simulink model "model_5modes"  (R2020a)
settings: Solver=VariableStepAuto  StartTime=0.0  StopTime=Inf  RelTol=1e-3
libraries: dspobslib x1
settings Model: Creator=Dinh-Viet-Toan  LastModifiedBy=Dinh-Viet-Toan

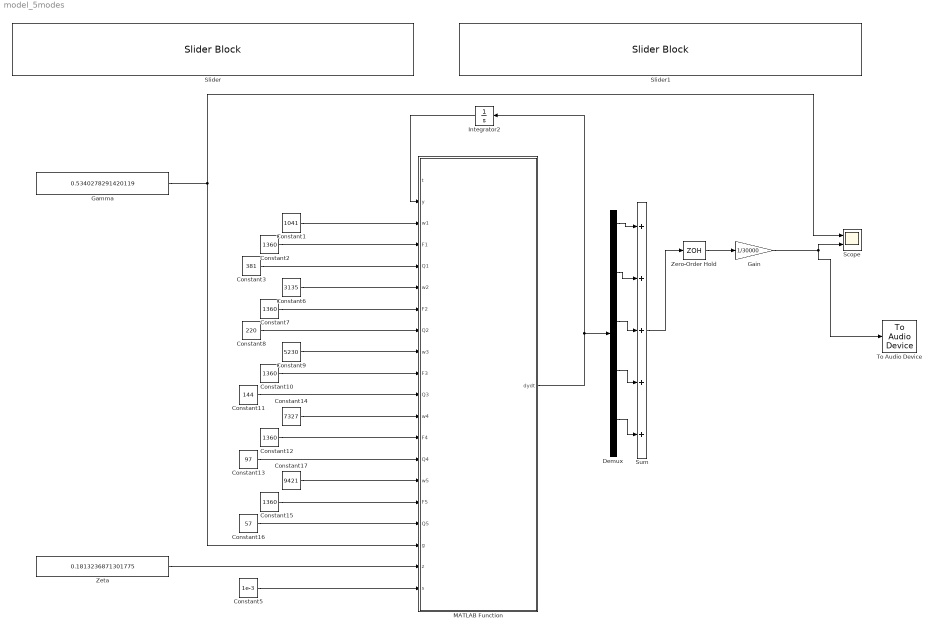
== system model_5modes ==
  Constant1 : Constant  Value=1041
  Constant{2,7,10,12,15} (5 alike) : Constant  Value=1360
  Constant11 : Constant  Value=144
  Constant13 : Constant  Value=97
  Constant14 : Constant  Value=7327
  Constant16 : Constant  Value=57
  Constant17 : Constant  Value=9421
  Constant3 : Constant  Value=381
  Constant5 : Constant  Value=1e-3
  Constant6 : Constant  Value=3135
  Constant8 : Constant  Value=220
  Constant9 : Constant  Value=5230
  Demux : Demux  Outputs=10
  Gain : Gain  Gain=1/30000
  Gamma : Constant  Value=0.5340278291420119
  Integrator2 : Integrator  InitialCondition=[0.01,0,0.01,0,0.01,0,0.01,0,0.01,0]
  MATLAB Function : MATLAB Function  TreatAsAtomicUnit=on
  Scope : Scope  NumInputPorts=2
  Slider : SliderBlock  ScaleMin=0.001  ScaleMax=1
  Slider1 : SliderBlock  ScaleMin=0.001  ScaleMax=1
  Sum : Sum  Inputs=+++++
  To Audio Device : dspobslib/To Audio Device  deviceName=Default  inheritSampleRate=off  sampleRate=44100  deviceDatatype=Determine from input data type  autoBufferSize=on  bufferSize=4096  queueDuration=1.0  defaultOutputChannelMapping=on  outputChannelMapping=1:2  outputNumUnderrunSamples=off
      settings: SourceProductBaseCode=DS
  Zero-Order Hold : ZeroOrderHold  SampleTime=1/22050
  Zeta : Constant  Value=0.1813236871301775
  wires:
  Gamma/1 -> MATLAB Function/18(g), Scope/1
  Zero-Order Hold/1 -> Gain/1
  Gain/1 -> To Audio Device/1, Scope/2
  Constant1/1 -> MATLAB Function/3(w1)
  Constant2/1 -> MATLAB Function/4(F1)
  Constant3/1 -> MATLAB Function/5(Q1)
  Integrator2/1 -> MATLAB Function/2(y)
  Zeta/1 -> MATLAB Function/19(z)
  Constant5/1 -> MATLAB Function/20(s)
  MATLAB Function/1(dydt) -> Integrator2/1, Demux/1
  Constant6/1 -> MATLAB Function/6(w2)
  Constant7/1 -> MATLAB Function/7(F2)
  Constant8/1 -> MATLAB Function/8(Q2)
  Constant9/1 -> MATLAB Function/9(w3)
  Constant10/1 -> MATLAB Function/10(F3)
  Constant11/1 -> MATLAB Function/11(Q3)
  Sum/1 -> Zero-Order Hold/1
  Demux/1 -> Sum/1
  Demux/3 -> Sum/2
  Demux/5 -> Sum/3
  Constant14/1 -> MATLAB Function/12(w4)
  Constant12/1 -> MATLAB Function/13(F4)
  Constant13/1 -> MATLAB Function/14(Q4)
  Constant17/1 -> MATLAB Function/15(w5)
  Constant15/1 -> MATLAB Function/16(F5)
  Constant16/1 -> MATLAB Function/17(Q5)
  Demux/7 -> Sum/4
  Demux/9 -> Sum/5

== matlab function model_5modes/MATLAB Function ==
  data: t input; dydt output; y input; w1 input; F1 input; Q1 input; w2 input; F2 input; Q2 input; w3 input; F3 input; Q3 input; w4 input; F4 input; Q4 input; w5 input; F5 input; Q5 input; g input; z input; s input
function dydt = systdyn_5modes(t,y,w1,F1,Q1,w2,F2,Q2,w3,F3,Q3,w4,F4,Q4,w5,F5,Q5,g,z,s)

dudt = ((y(2) + y(4) + y(6) + y(8) + y(10))*z*(g - y(1) - y(3) - y(5) - y(7) - y(9)))/(s + (g - y(1) - y(3) - y(5) - y(7) - y(9))^2)^(1/4) + ((-y(2) - y(4) - y(6) - y(8) - y(10))*z*(1 - g + y(1) + y(3) + y(5) + y(7) + y(9)))/(s + (g - y(1) - y(3) - y(5) - y(7) - y(9))^2)^(1/4) - ((-y(2) - y(4) - y(6) - y(8) - y(10))*z*(g - y(1) - y(3) - y(5) - y(7) - y(9))^2*(1 - g + y(1) + y(3) + y(5) + y(7) + y(9)))/(2*(s + (g - y(1) - y(3) - y(5) - y(7) - y(9))^2)^(5/4));

% dudt = ((y(2) + y(4) + y(6))*z*(g - y(1) - y(3) - y(5)))/(s + (g - y(1) - y(3) - y(5))^2)^(1/4) + ((-y(2) - y(4) - y(6))*z*(1 - g + y(1) + y(3) + y(5)))/(s + (g - y(1) - y(3) - y(5))^2)^(1/4) - ((-y(2) - y(4) - y(6))*z*(g - y(1) - y(3) - y(5))^2*(1 - g + y(1) + y(3) + y(5)))/(2*(s + (g - y(1) - y(3) - y(5))^2)^(5/4));
% Ecriture vectorielle Y'=F(Y)

dydt1 = [y(2); -(w1/Q1)*y(2) - w1^2*y(1) + F1*dudt];
dydt2 = [y(4); -(w2/Q2)*y(4) - w2^2*y(3) + F2*dudt];
dydt3 = [y(6); -(w3/Q3)*y(6) - w3^2*y(5) + F3*dudt];
dydt4 = [y(8); -(w4/Q4)*y(8) - w4^2*y(7) + F4*dudt];
dydt5 = [y(10); -(w5/Q5)*y(10) - w5^2*y(9) + F5*dudt];

dydt = [dydt1;dydt2;dydt3;dydt4;dydt5];
end
